simulink model "dcm_dc"  (R2017b)
settings: Solver=ode45  StartTime=0.0  StopTime=1  RelTol=1e-6  AbsTol=1e-6  EnableMultiTasking=on
values from neighbouring files (symbols this model uses):
  D = 0.002    [task1.m]
  J = 0.05    [task1.m]
  La = 0.03    [task1.m]
  psim = 1.1    [task1.m]
  Ra = 3    [task1.m]
  U = 100    [task1.m]
settings Model: Creator=ielolof  LastModifiedBy=Morten
settings DataIOCC: LimitDataPoints=on  SaveFormat=Array  SignalLoggingSaveFormat=ModelDataLogs  TimeSaveName=tdc
settings OptimizationCC: ExpressionDepthLimit=2147483647  InitFltsAndDblsToZero=on  LifeSpan=inf
settings DebuggingCC: UnderspecifiedInitializationDetection=Classic  MergeDetectMultiDrivingBlocksExec=none  SolverPrmCheckMsg=warning  FcnCallInpInsideContextMsg=warning  StateNameClashWarn=warning  StrictBusMsg=Warning  SFUnexpectedBacktrackingDiag=warning  SFNoUnconditionalDefaultTransitionDiag=warning  SFExecutionAtInitializationDiag=none
settings HardwareCC: ProdBitPerPointer=32  ProdBitPerSizeT=32  ProdBitPerPtrDiffT=32  ProdLargestAtomicFloat=None  ProdIntDivRoundTo=Undefined  ProdEndianess=Unspecified  ProdWordSize=32  ProdHWDeviceType=32-bit Generic
settings ModelReferenceCC: PropagateSignalLabelsOutOfModel=off
settings CodeAppCC: StateflowObjectComments=on
settings GRTTargetCC: TargetLangStandard=C89/C90 (ANSI)  CombineOutputUpdateFcns=off  GRTInterface=on
settings ConfigComp: CovMetricSettings=dw  CovHtmlReporting=on  CovSaveCumulativeToWorkspaceVar=on  CovSaveSingleToWorkspaceVar=on  CovExternalEMLEnable=off

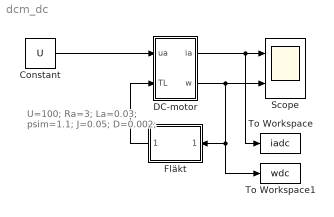
== system dcm_dc ==
  note: U=100;
      | Ra=3;
      | La=0.03;
      | psim=1.1;
      | J=0.05;
      | D=0.002;
  Constant : Constant  Value=U
  DC-motor : Subsystem
  Fläkt : Subsystem
  Scope : Scope  NumInputPorts=2
  To Workspace : ToWorkspace  VariableName=iadc  SampleTime=-1
  To Workspace1 : ToWorkspace  VariableName=wdc  SampleTime=-1
  wires:
  Constant/1 -> DC-motor/1(ua)
  DC-motor/1(ia) -> Scope/1, To Workspace/1
  DC-motor/2(w) -> Scope/2, Fläkt/1(wfan), To Workspace1/1
  Fläkt/1(Tfan) -> DC-motor/2(TL)

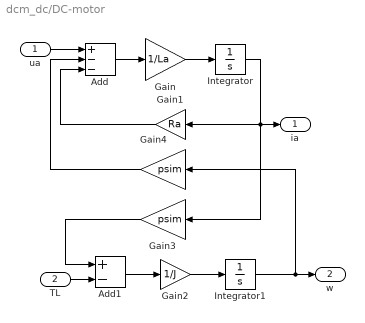
== system dcm_dc/DC-motor ==
  ua : Inport
  TL : Inport  Port=2
  Add : Sum  Inputs=+--
  Add1 : Sum  Inputs=+-
  Gain : Gain  Gain=1/La
  Gain1 : Gain  Gain=Ra
  Gain2 : Gain  Gain=1/J
  Gain3 : Gain  Gain=psim
  Gain4 : Gain  Gain=psim
  Integrator : Integrator
  Integrator1 : Integrator
  ia : Outport
  w : Outport  Port=2
  wires:
  Add/1 -> Gain/1
  Gain/1 -> Integrator/1
  Integrator/1 -> Gain1/1, Gain3/1, ia/1
  Add1/1 -> Gain2/1
  Gain2/1 -> Integrator1/1
  Gain3/1 -> Add1/1
  Integrator1/1 -> w/1, Gain4/1
  Gain1/1 -> Add/3
  Gain4/1 -> Add/2
  ua/1 -> Add/1
  TL/1 -> Add1/2

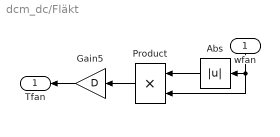
== system dcm_dc/Fläkt ==
  wfan : Inport
  Abs : Abs
  Gain5 : Gain  Gain=D
  Product : Product  RndMeth=Zero
  Tfan : Outport
  wires:
  Product/1 -> Gain5/1
  Abs/1 -> Product/1
  wfan/1 -> Abs/1, Product/2
  Gain5/1 -> Tfan/1
